simulink model "sim_red_ad_lgr"  (R2020b)
settings: Solver=VariableStepAuto  StartTime=0.0  StopTime=36  RelTol=1e-3
values from neighbouring files (symbols this model uses):
  k = 1.05    [lgr_atraso.m]    (also in lgr_atraso_adelanto.m = 1/div)
  p = 0.005    [lgr_atraso.m]
  z = p*10    (= 0.05)    [lgr_atraso.m]
libraries: simulink x1
settings Model: Creator=Acer  LastModifiedBy=Acer

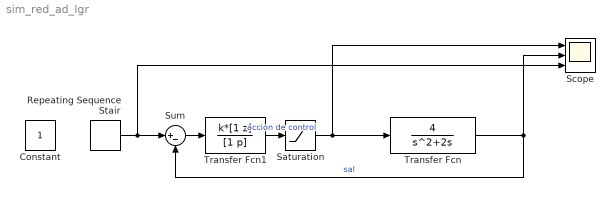
== system sim_red_ad_lgr ==
  Constant : Constant  SampleTime=6
  Repeating Sequence Stair : simulink/Sources/Repeating Sequence Stair  OutValues=[1 -0.5 2 5 -2.5].'  tsamp=6  OutMin=[]  OutMax=[]  OutDataTypeStr=double  OutputDataTypeScalingMode=double  OutDataType=fixdt(0,8)  ConRadixGroup=Best Precision: Vector-wise  OutScaling=2^-12
  Saturation : Saturate  UpperLimit=13  LowerLimit=-13
  Scope : Scope  NumInputPorts=3
  Sum : Sum  Inputs=|+-
  Transfer Fcn : TransferFcn  Numerator=[4]  Denominator=[1 2 0]
  Transfer Fcn1 : TransferFcn  Numerator=k*[1 z]  Denominator=[1 p]
  wires:
  Transfer Fcn1/1 -> Saturation/1  "accion de control"
  Transfer Fcn/1 -> Scope/2, Sum/2  "sal"
  Sum/1 -> Transfer Fcn1/1
  Repeating Sequence Stair/1 -> Scope/3, Sum/1
  Saturation/1 -> Transfer Fcn/1, Scope/1
